simulink model "Simulatore_analogico_rev3"  (Simulink 7.7)
settings: Solver=ode3  StartTime=0.0  StopTime=stop_t  FixedStep=Ts  MaxStep=Ts/10  MinStep=Ts/100  RelTol=1e-3
values from neighbouring files (symbols this model uses):
  a_da = 0    [CA_GIUSE.m]    (also in Script.m)
  a_dp = 0e-2    (= 0)    [CA_GIUSE.m]    (also in Script.m)
  a_ds = 0e-2    (= 0)    [CA_GIUSE.m]    (also in Script.m)
  aph = 0.00    (= 0)    [CA_GIUSE.m]    (also in Script.m = 0.05)
  Da_c = 0e-3    (= 0)    [CA_GIUSE.m]    (also in Script.m)
  Da_r = 0    [CA_GIUSE.m]    (also in Script.m)
  Dp_c = 0e-4    (= 0)    [CA_GIUSE.m]    (also in Script.m)
  Dp_r = 0    [CA_GIUSE.m]    (also in Script.m)
  Ds_c = 0    [CA_GIUSE.m]    (also in Script.m)
  Ds_r = 0    [CA_GIUSE.m]    (also in Script.m)
  Ga = 0e3    (= 0)    [CA_GIUSE.m]    (also in Script.m)
  Gdp = 0    [CA_GIUSE.m]    (also in Script.m = 1)
  Gf = 1/(Kd*Gs)    [CA_GIUSE.m]    (also in Script.m)
  Gr = 0    [CA_GIUSE.m]    (also in Script.m = 1)
  Gs =     [CA_GIUSE.m]    (also in Script.m = 0)
  Kd =     [CA_GIUSE.m]    (also in Script.m = 0)
  over = 0.0    (= 0)    [CA_GIUSE.m]    (also in Script.m)
  Pulse_da = 0    [CA_GIUSE.m]    (also in Script.m)
  Pulse_dp = 0e-0    (= 0)    [CA_GIUSE.m]    (also in Script.m)
  Pulse_ds = 0    [CA_GIUSE.m]    (also in Script.m)
  R_0 = 1    [CA_GIUSE.m]    (also in Script.m)
undefined symbols (not defined in the file or in its folder): den_Gc, den_Gp, num_Gc, num_Gp
libraries: simulink x18
settings Model: Creator=Sandro  LastModifiedBy=giuse

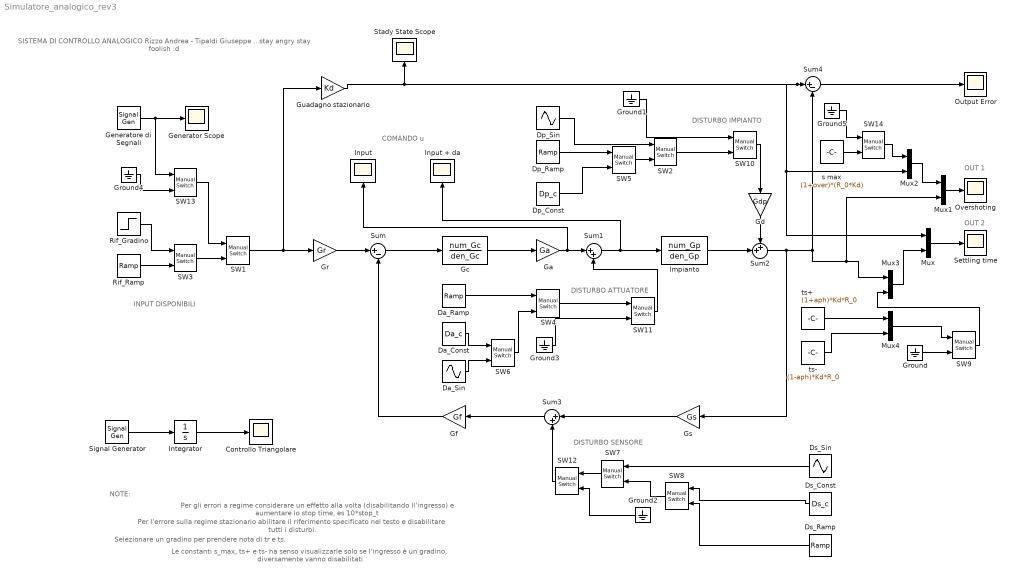
== system Simulatore_analogico_rev3 ==
  note: SISTEMA DI CONTROLLO ANALOGICO
      | Rizzo Andrea - Tipaldi Giuseppe
      |
      | ...stay angry stay foolish
      | :d
  note: DISTURBO ATTUATORE
  note: DISTURBO IMPIANTO
  note: INPUT DISPONIBILI
  note: COMANDO u
  note: DISTURBO SENSORE
  note: OUT 1
  note: OUT 2
  note: NOTE:
  note: Per gli errori a regime considerare un effetto alla volta (disabilitando ll'ingresso) e aumentare lo stop time, es 10*stop_t
  note: Selezionare un gradino per prendere nota di tr e ts.
  note: Per l'errore sulla regime stazionario abilitare il riferimento specificato nel testo e disabilitare tutti i disturbi.
  note: Le constanti s_max, ts+ e ts- ha senso visualizzarle solo se l'ingresso è un gradino, diversamente vanno disabilitati
  " s max" : Constant  Value=(1+over)*(R_0*Kd)
  Controllo Triangolare : Scope
      settings: SaveName=ScopeData3
  Da_Const : Constant  Value=Da_c
  Da_Ramp : simulink/Sources/Ramp  SystemSampleTime=-1  slope=Da_r  start=0  X0=0
  Da_Sin : Sin  Amplitude=a_da  Frequency=Pulse_da  SampleTime=0
  Dp_Const : Constant  Value=Dp_c
  Dp_Ramp : simulink/Sources/Ramp  SystemSampleTime=-1  slope=Dp_r  start=0  X0=0
  Dp_Sin : Sin  Amplitude=a_dp  Frequency=Pulse_dp  SampleTime=0
  Ds_Const : Constant  Value=Ds_c
  Ds_Ramp : simulink/Sources/Ramp  SystemSampleTime=-1  slope=Ds_r  start=0  X0=0
  Ds_Sin : Sin  Amplitude=a_ds  Frequency=Pulse_ds  SampleTime=0
  Ga : Gain  Gain=Ga
  Gc : TransferFcn  Numerator=num_Gc  Denominator=den_Gc
  Gd : Gain  Gain=Gdp
  Generator Scope : Scope
      settings: TimeRange=0.002216033935546875  YMin=2.1909418072197  YMax=2.191153294711311  SaveName=ScopeData6
  Generatore di Segnali : SignalGenerator  WaveForm=square  Amplitude=0.1  Frequency=0.25
  Gf : Gain  Gain=Gf
  Gr : Gain  Gain=Gr
  Ground{,1..5} (6 alike) : Ground
  Gs : Gain  Gain=Gs
  Guadagno stazionario : Gain  Gain=Kd
  Impianto : TransferFcn  Numerator=num_Gp  Denominator=den_Gp
  Input : Scope
      settings: TimeRange=7.62942779291553  YMin=0.9536585365853658  YMax=1.036585365853659  SaveName=ScopeData4
  Input + da : Scope
      settings: TimeRange=7.62942779291553  YMin=0.9536585365853658  YMax=1.036585365853659
  Integrator : Integrator  InitialCondition=0.5
  Mux{,1..4} (5 alike) : Mux  Inputs=2
  Output Error : Scope
      settings: TimeRange=25  YMin=-0.0003150000000000001  YMax=0.0001950000000000001  SaveName=ScopeData2
  Overshoting : Scope
      settings: TimeRange=0.002216033935546875  YMin=0.000179875  YMax=0.0001802  SaveName=ScopeData5
  Rif_Gradino : Step  Time=0  After=R_0  SampleTime=0
  Rif_Ramp : simulink/Sources/Ramp  SystemSampleTime=-1  slope=R_0  start=0  X0=0
  SW{1,4,9,11..12,14} (6 alike) : simulink/Signal Routing/Manual Switch  SystemSampleTime=-1  sw=0  action=0  varsize=off
  SW{2..3,5..8,10,13} (8 alike) : simulink/Signal Routing/Manual Switch  SystemSampleTime=-1  sw=1  action=0  varsize=off
  Settling time : Scope
      settings: TimeRange=10  YMin=0  YMax=3.5
  Signal Generator : SignalGenerator  WaveForm=square  Amplitude=0.5  Frequency=0.25
  Stady State Scope : Scope
      settings: TimeRange=7.62942779291553  YMin=0.9536585365853658  YMax=1.036585365853659  SaveName=ScopeData7
  Sum : Sum  Inputs=|+-
  Sum1 : Sum  Inputs=|++
  Sum2 : Sum  Inputs=++|
  Sum3 : Sum  Inputs=|++
  Sum4 : Sum  Inputs=|+-
  ts+ : Constant  Value=(1+aph)*Kd*R_0
  ts- : Constant  Value=(1-aph)*Kd*R_0
  wires:
  Sum1/1 -> Impianto/1, Input + da/1
  Sum2/1 -> Gs/1, Mux3/1, Mux1/2, Sum4/2
  Ga/1 -> Sum1/1, Input/1
  Guadagno stazionario/1 -> Sum4/1, Mux/1, Mux2/2, Stady State Scope/1
  Mux/1 -> Settling time/1
  Signal Generator/1 -> Integrator/1
  Impianto/1 -> Sum2/2
  Gd/1 -> Sum2/1
  Gs/1 -> Sum3/1
  Gr/1 -> Sum/1
  SW3/1 -> SW1/2
  SW5/1 -> SW2/2
  SW6/1 -> SW4/2
  Dp_Const/1 -> SW5/2
  Dp_Sin/1 -> SW2/1
  Dp_Ramp/1 -> SW5/1
  Da_Sin/1 -> SW6/2
  Da_Const/1 -> SW6/1
  Da_Ramp/1 -> SW4/1
  Rif_Ramp/1 -> SW3/2
  Rif_Gradino/1 -> SW3/1
  SW8/1 -> SW7/2
  Ds_Sin/1 -> SW7/1
  Ds_Const/1 -> SW8/1
  Ds_Ramp/1 -> SW8/2
  Sum4/1 -> Output Error/1
  ts-/1 -> Mux4/2
  ts+/1 -> Mux4/1
  Mux4/1 -> SW9/1
  SW9/1 -> Mux3/2
  Ground/1 -> SW9/2
  Mux1/1 -> Overshoting/1
  SW2/1 -> SW10/2
  SW10/1 -> Gd/1
  Ground1/1 -> SW10/1
  SW7/1 -> SW12/1
  SW12/1 -> Sum3/2
  Ground2/1 -> SW12/2
  SW4/1 -> SW11/1
  Ground3/1 -> SW11/2
  SW11/1 -> Sum1/2
  SW13/1 -> SW1/1
  Generatore di Segnali/1 -> SW13/1, Generator Scope/1
  Ground4/1 -> SW13/2
  Mux3/1 -> Mux/2
  Integrator/1 -> Controllo Triangolare/1
  SW1/1 -> Gr/1, Guadagno stazionario/1
  Sum3/1 -> Gf/1
  Gf/1 -> Sum/2
  Mux2/1 -> Mux1/1
  " s max"/1 -> SW14/2
  SW14/1 -> Mux2/1
  Ground5/1 -> SW14/1
  Sum/1 -> Gc/1
  Gc/1 -> Ga/1
